simulink model "ZSPARK"  (R2026a)
settings: Solver=ode45  StopTime=0.010  FixedStep=1e-6
libraries: commrandsrc3 x5
settings Model: Creator=SANDESH  LastModifiedBy=SANDESH

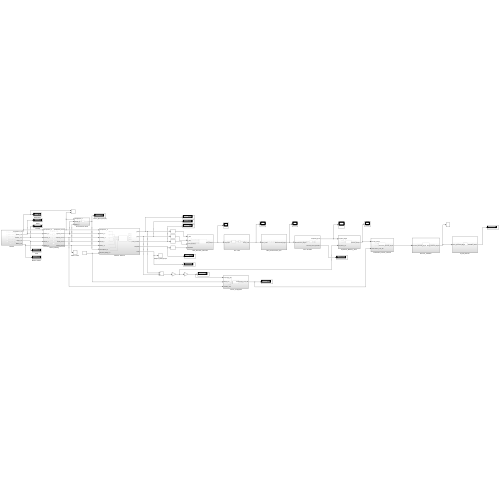
[thumbnail: Simulink's stored preview of the top-level diagram]
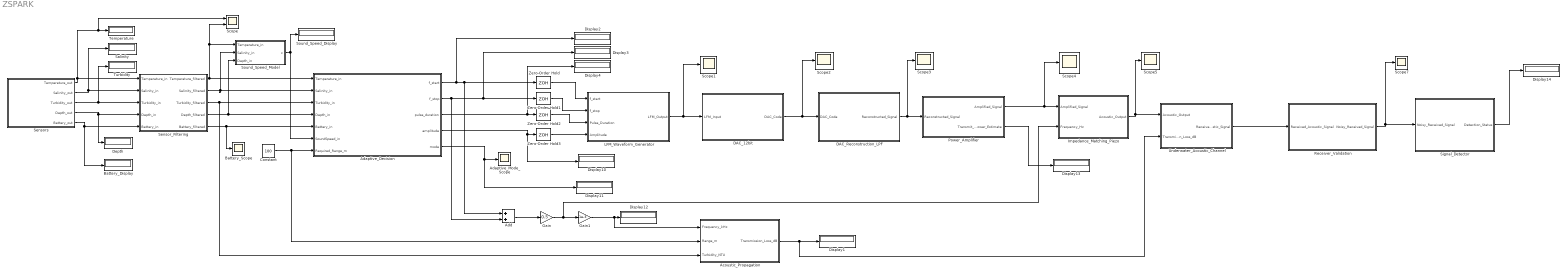
== system ZSPARK ==
  Acoustic_Propagation : Subsystem
  Adaptive_Decision : Subsystem
  Adaptive_Mode_Scope : Scope
      settings: TimeSpan=2  ActiveDisplayYMinimum=3  ActiveDisplayYMaximum=5  DataLoggingVariableName=ScopeData7
  Add : Sum
  Battery_Display : Display
  Battery_Scope : Scope
      settings: ActiveDisplayYMinimum=10.05  ActiveDisplayYMaximum=30.05  DataLoggingVariableName=ScopeData8
  Constant : Constant  Value=100
  DAC_12bit : Subsystem
  DAC_Reconstruction_LPF : Subsystem
  "Depth " : Display
  Display{1..4,10..14} (9 alike) : Display
  Gain : Gain  Gain=0.5
  Gain1 : Gain  Gain=1e-3
  Impedance_Matching_Piezo : Subsystem
  LFM_Waveform_Generator : Subsystem
  Power_Amplifier : Subsystem
  Receiver_Validation : Subsystem
  Salinity : Display
  Scope : Scope  NumInputPorts=2
      settings: TimeSpan=5  ActiveDisplayYMinimum=24.73062316838924  ActiveDisplayYMaximum=25.037041154016777
  Scope{1..5,7} (6 alike) : Scope
      Scope1 settings: TimeSpan=0.01  ActiveDisplayYMinimum=-1.0116208794215797  ActiveDisplayYMaximum=0.70243286352046441  DataLoggingDecimation=10
      Scope2 settings: TimeSpan=5e-3  ActiveDisplayYMinimum=1213.15  ActiveDisplayYMaximum=2904.4  DataLoggingVariableName=ScopeData2
      Scope3 settings: ActiveDisplayYMinimum=-0.37290125281823788  ActiveDisplayYMaximum=0.44819314690823536  DataLoggingVariableName=ScopeData3
      Scope4 settings: ActiveDisplayYMinimum=-0.82095317211603991  ActiveDisplayYMaximum=0.82123562733690658  DataLoggingVariableName=ScopeData4
      Scope5 settings: ActiveDisplayYMinimum=-0.38776131013108261  ActiveDisplayYMaximum=0.42690430214579189  DataLoggingVariableName=ScopeData5
      Scope7 settings: TimeSpan=0.01  ActiveDisplayYMinimum=-0.00440701448520266  ActiveDisplayYMaximum=0.0042196253860243855  DataLoggingVariableName=ScopeData9
  Sensor_Filtering : Subsystem
  Sensors : Subsystem
  Signal_Detector : Subsystem
  Sound_Speed_Display : Display
  Sound_Speed_Model : Subsystem
  "Temperature " : Display
  Turbidity : Display
  Underwater_Acoustic_Channel : Subsystem
  Zero-Order Hold{,1..3} (4 alike) : ZeroOrderHold  SampleTime=1e-6
  wires:
  Sensors/5(Battery_out) -> Sensor_Filtering/5(Battery_in), Battery_Display/1
  Sensors/4(Depth_out) -> Sensor_Filtering/4(Depth_in), "Depth "/1
  Sensors/2(Salinity_out) -> Sensor_Filtering/2(Salinity_in), Salinity/1
  Sensors/3("Turbidity_out ") -> Sensor_Filtering/3("Turbidity_in "), Turbidity/1
  Sensors/1(Temperature_out) -> Sensor_Filtering/1(Temperature_in), Scope/1, "Temperature "/1
  Sensor_Filtering/1(Temperature_filtered) -> Scope/2, Sound_Speed_Model/1(Temperature_in), Adaptive_Decision/1(Temperature_in)
  Sensor_Filtering/2(Salinity_filtered) -> Sound_Speed_Model/2(Salinity_in), Adaptive_Decision/2(Salinity_in)
  Sensor_Filtering/4(Depth_filtered) -> Sound_Speed_Model/3(Depth_in), Adaptive_Decision/4(Depth_in)
  Sound_Speed_Model/1(c) -> Adaptive_Decision/6(SoundSpeed_in), Sound_Speed_Display/1
  Gain1/1 -> Acoustic_Propagation/1(Frequency_kHz), Display12/1
  Constant/1 -> Acoustic_Propagation/2(Range_m), Adaptive_Decision/7(Required_Range_m)
  Sensor_Filtering/3(Turbidity_filtered) -> Acoustic_Propagation/3(Turbidity_NTU), Adaptive_Decision/3("Turbidity_in ")
  Sensor_Filtering/5(Battery_filtered) -> Battery_Scope/1, Adaptive_Decision/5(Battery_in)
  Adaptive_Decision/1(f_start) -> Display2/1, Add/1, Zero-Order Hold/1
  Adaptive_Decision/2(f_stop) -> Add/2, Zero-Order Hold1/1, Display3/1
  Adaptive_Decision/3(pulse_duration) -> Display4/1, Zero-Order Hold2/1
  Adaptive_Decision/5(mode) -> Display11/1, Adaptive_Mode_Scope/1
  Gain/1 -> Impedance_Matching_Piezo/2(Frequency_Hz), Gain1/1
  LFM_Waveform_Generator/1(LFM_Output) -> Scope1/1, DAC_12bit/1(LFM_Input)
  Zero-Order Hold/1 -> LFM_Waveform_Generator/1(f_start)
  Zero-Order Hold1/1 -> LFM_Waveform_Generator/2(f_stop)
  Zero-Order Hold3/1 -> LFM_Waveform_Generator/4(Amplitude)
  Zero-Order Hold2/1 -> LFM_Waveform_Generator/3(Pulse_Duration)
  DAC_12bit/1(DAC_Code) -> Scope2/1, DAC_Reconstruction_LPF/1(DAC_Code)
  DAC_Reconstruction_LPF/1(Reconstructed_Signal) -> Power_Amplifier/1(Reconstructed_Signal), Scope3/1
  Power_Amplifier/1(Amplified_Signal) -> Impedance_Matching_Piezo/1(Amplified_Signal), Scope4/1
  Power_Amplifier/2(Transmit_Power_Estimate) -> Display13/1
  Impedance_Matching_Piezo/1(Acoustic_Output) -> Scope5/1, Underwater_Acoustic_Channel/1(Acoustic_Output)
  Adaptive_Decision/4(amplitude) -> Display10/1, Zero-Order Hold3/1
  Add/1 -> Gain/1
  Underwater_Acoustic_Channel/1(Received_Acoustic_Signal) -> Receiver_Validation/1(Received_Acoustic_Signal)
  Acoustic_Propagation/1(Transmission_Loss_dB) -> Underwater_Acoustic_Channel/2(Transmission_Loss_dB), Display1/1
  Receiver_Validation/1(Noisy_Received_Signal) -> Signal_Detector/1(Noisy_Received_Signal), Scope7/1
  Signal_Detector/1(Detection_Status) -> Display14/1

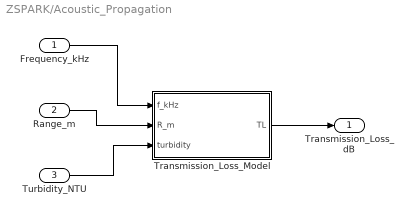
== system ZSPARK/Acoustic_Propagation ==
  Frequency_kHz : Inport
  Range_m : Inport  Port=2
  Turbidity_NTU : Inport  Port=3
  Transmission_Loss_Model : MATLAB Function  TreatAsAtomicUnit=on
  Transmission_Loss_dB : Outport
  wires:
  Frequency_kHz/1 -> Transmission_Loss_Model/1(f_kHz)
  Range_m/1 -> Transmission_Loss_Model/2(R_m)
  Turbidity_NTU/1 -> Transmission_Loss_Model/3(turbidity)
  Transmission_Loss_Model/1(TL) -> Transmission_Loss_dB/1

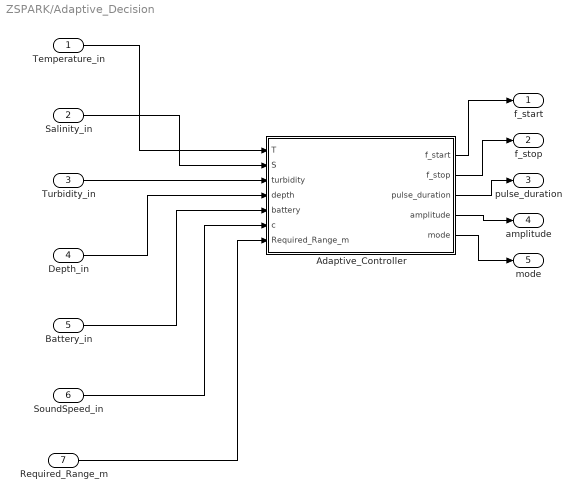
== system ZSPARK/Adaptive_Decision ==
  Temperature_in : Inport
  Salinity_in : Inport  Port=2
  "Turbidity_in " : Inport  Port=3
  Depth_in : Inport  Port=4
  Battery_in : Inport  Port=5
  SoundSpeed_in : Inport  Port=6
  Required_Range_m : Inport  Port=7
  Adaptive_Controller : MATLAB Function  TreatAsAtomicUnit=on
  f_start : Outport
  f_stop : Outport  Port=2
  pulse_duration : Outport  Port=3
  amplitude : Outport  Port=4
  mode : Outport  Port=5
  wires:
  Battery_in/1 -> Adaptive_Controller/5(battery)
  "Turbidity_in "/1 -> Adaptive_Controller/3(turbidity)
  Salinity_in/1 -> Adaptive_Controller/2(S)
  Temperature_in/1 -> Adaptive_Controller/1(T)
  Depth_in/1 -> Adaptive_Controller/4(depth)
  SoundSpeed_in/1 -> Adaptive_Controller/6(c)
  Adaptive_Controller/5(mode) -> mode/1
  Adaptive_Controller/4(amplitude) -> amplitude/1
  Adaptive_Controller/3(pulse_duration) -> pulse_duration/1
  Adaptive_Controller/2(f_stop) -> f_stop/1
  Adaptive_Controller/1(f_start) -> f_start/1
  Required_Range_m/1 -> Adaptive_Controller/7(Required_Range_m)

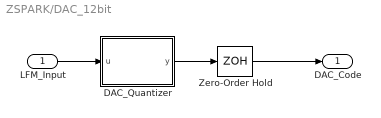
== system ZSPARK/DAC_12bit ==
  LFM_Input : Inport
  DAC_Quantizer : MATLAB Function  TreatAsAtomicUnit=on
  Zero-Order Hold : ZeroOrderHold  SampleTime=-1
  DAC_Code : Outport
  wires:
  LFM_Input/1 -> DAC_Quantizer/1(u)
  DAC_Quantizer/1(y) -> Zero-Order Hold/1
  Zero-Order Hold/1 -> DAC_Code/1

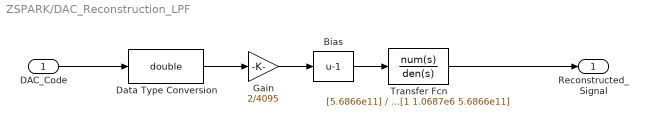
== system ZSPARK/DAC_Reconstruction_LPF ==
  DAC_Code : Inport
  Bias : Bias  Bias=-1  SaturateOnIntegerOverflow=off
  Data Type Conversion : DataTypeConversion  OutDataTypeStr=double  SaturateOnIntegerOverflow=off  RndMeth=Floor
  Gain : Gain  Gain=2/4095
  Transfer Fcn : TransferFcn  Numerator=[5.6866e11]  Denominator=[1 1.0687e6 5.6866e11]
  Reconstructed_Signal : Outport
  wires:
  DAC_Code/1 -> Data Type Conversion/1
  Data Type Conversion/1 -> Gain/1
  Gain/1 -> Bias/1
  Bias/1 -> Transfer Fcn/1
  Transfer Fcn/1 -> Reconstructed_Signal/1

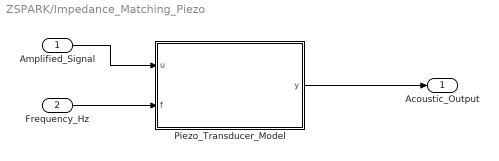
== system ZSPARK/Impedance_Matching_Piezo ==
  Amplified_Signal : Inport
  Frequency_Hz : Inport  Port=2
  Piezo_Transducer_Model : MATLAB Function  TreatAsAtomicUnit=on
  Acoustic_Output : Outport
  wires:
  Frequency_Hz/1 -> Piezo_Transducer_Model/2(f)
  Amplified_Signal/1 -> Piezo_Transducer_Model/1(u)
  Piezo_Transducer_Model/1(y) -> Acoustic_Output/1

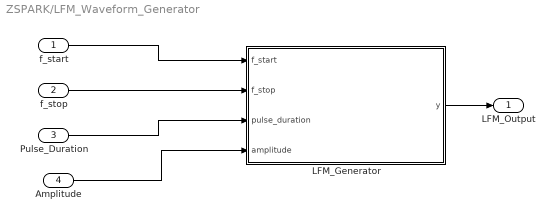
== system ZSPARK/LFM_Waveform_Generator ==
  f_start : Inport
  f_stop : Inport  Port=2
  Pulse_Duration : Inport  Port=3
  Amplitude : Inport  Port=4
  LFM_Generator : MATLAB Function  TreatAsAtomicUnit=on
  LFM_Output : Outport
  wires:
  f_start/1 -> LFM_Generator/1(f_start)
  f_stop/1 -> LFM_Generator/2(f_stop)
  Pulse_Duration/1 -> LFM_Generator/3(pulse_duration)
  Amplitude/1 -> LFM_Generator/4(amplitude)
  LFM_Generator/1(y) -> LFM_Output/1

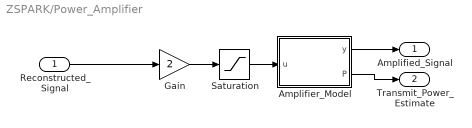
== system ZSPARK/Power_Amplifier ==
  Reconstructed_Signal : Inport
  Amplifier_Model : MATLAB Function  TreatAsAtomicUnit=on
  Gain : Gain  Gain=2
  Saturation : Saturate  UpperLimit=1  LowerLimit=-1
  Amplified_Signal : Outport
  Transmit_Power_Estimate : Outport  Port=2
  wires:
  Reconstructed_Signal/1 -> Gain/1
  Gain/1 -> Saturation/1
  Saturation/1 -> Amplifier_Model/1(u)
  Amplifier_Model/1(y) -> Amplified_Signal/1
  Amplifier_Model/2(P) -> Transmit_Power_Estimate/1

== system ZSPARK/Receiver_Validation ==
  Received_Acoustic_Signal : Inport
  Underwater_Noise_Model : MATLAB Function  TreatAsAtomicUnit=on
  Noisy_Received_Signal : Outport
  wires:
  Received_Acoustic_Signal/1 -> Underwater_Noise_Model/1(u)
  Underwater_Noise_Model/1(y) -> Noisy_Received_Signal/1

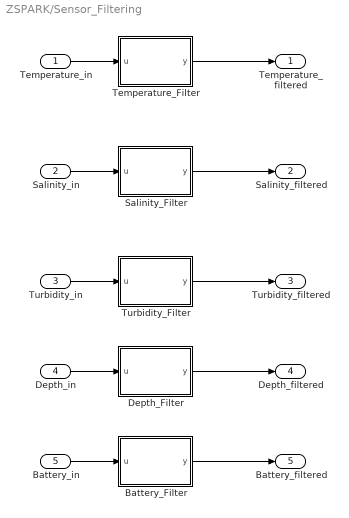
== system ZSPARK/Sensor_Filtering ==
  Temperature_in : Inport
  Salinity_in : Inport  Port=2
  "Turbidity_in " : Inport  Port=3
  Depth_in : Inport  Port=4
  Battery_in : Inport  Port=5
  Battery_Filter : MATLAB Function  TreatAsAtomicUnit=on
  Depth_Filter : MATLAB Function  TreatAsAtomicUnit=on
  Salinity_Filter : MATLAB Function  TreatAsAtomicUnit=on
  "Temperature_Filter " : MATLAB Function  TreatAsAtomicUnit=on
  Turbidity_Filter : MATLAB Function  TreatAsAtomicUnit=on
  Temperature_filtered : Outport
  Salinity_filtered : Outport  Port=2
  Turbidity_filtered : Outport  Port=3
  Depth_filtered : Outport  Port=4
  Battery_filtered : Outport  Port=5
  wires:
  Temperature_in/1 -> "Temperature_Filter "/1(u)
  Salinity_in/1 -> Salinity_Filter/1(u)
  "Turbidity_in "/1 -> Turbidity_Filter/1(u)
  Depth_in/1 -> Depth_Filter/1(u)
  Battery_in/1 -> Battery_Filter/1(u)
  "Temperature_Filter "/1(y) -> Temperature_filtered/1
  Salinity_Filter/1(y) -> Salinity_filtered/1
  Turbidity_Filter/1(y) -> Turbidity_filtered/1
  Depth_Filter/1(y) -> Depth_filtered/1
  Battery_Filter/1(y) -> Battery_filtered/1

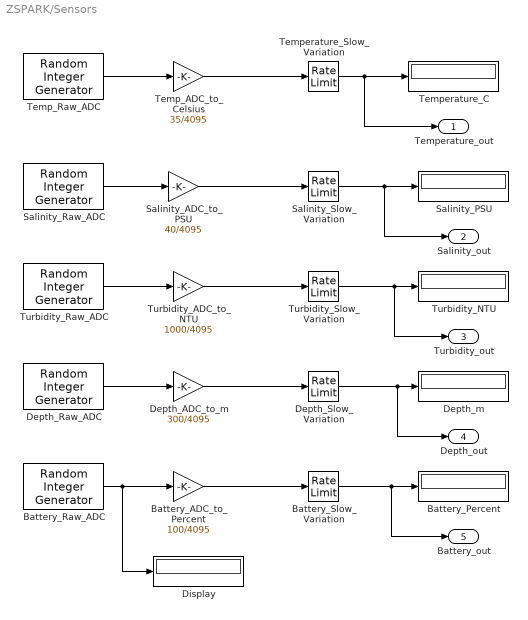
== system ZSPARK/Sensors ==
  Battery_ADC_to_Percent : Gain  Gain=100/4095
  Battery_Percent : Display
  Battery_Raw_ADC : commrandsrc3/Random Integer Generator  SetSize=4096  SeedSource=Parameter  Seed=56789  SampleTime=0.1  SamplesPerFrame=1  OutputDataType=double  SimulateUsing=Interpreted execution
  Battery_Slow_Variation : RateLimiter  RisingSlewLimit=0.5  FallingSlewLimit=-0.5  SampleTimeMode=inherited  InitialCondition=20
  Depth_ADC_to_m : Gain  Gain=300/4095
  Depth_Raw_ADC : commrandsrc3/Random Integer Generator  SetSize=2730  SeedSource=Parameter  Seed=45678  SampleTime=0.1  SamplesPerFrame=1  OutputDataType=double  SimulateUsing=Interpreted execution
  Depth_Slow_Variation : RateLimiter  RisingSlewLimit=2  FallingSlewLimit=-2  SampleTimeMode=inherited  InitialCondition=100
  Depth_m : Display
  Display : Display
  Salinity_ADC_to_PSU : Gain  Gain=40/4095
  Salinity_PSU : Display
  Salinity_Raw_ADC : commrandsrc3/Random Integer Generator  SetSize=4096  SeedSource=Parameter  Seed=23456  SampleTime=0.1  SamplesPerFrame=1  OutputDataType=double  SimulateUsing=Interpreted execution
  Salinity_Slow_Variation : RateLimiter  RisingSlewLimit=0.2  FallingSlewLimit=-0.2  SampleTimeMode=inherited  InitialCondition=35
  Temp_ADC_to_Celsius : Gain  Gain=35/4095
  Temp_Raw_ADC : commrandsrc3/Random Integer Generator  SetSize=4096  SeedSource=Parameter  Seed=12345  SampleTime=0.1  SamplesPerFrame=1  OutputDataType=double  SimulateUsing=Interpreted execution
  Temperature_C : Display
  Temperature_Slow_Variation : RateLimiter  RisingSlewLimit=0.2  FallingSlewLimit=-0.2  SampleTimeMode=inherited  InitialCondition=25
  Turbidity_ADC_to_NTU : Gain  Gain=1000/4095
  Turbidity_NTU : Display
  Turbidity_Raw_ADC : commrandsrc3/Random Integer Generator  SetSize=4096  SeedSource=Parameter  Seed=34567  SampleTime=0.1  SamplesPerFrame=1  OutputDataType=double  SimulateUsing=Interpreted execution
  Turbidity_Slow_Variation : RateLimiter  RisingSlewLimit=20  FallingSlewLimit=-20  SampleTimeMode=inherited  InitialCondition=500
  Temperature_out : Outport
  Salinity_out : Outport  Port=2
  "Turbidity_out " : Outport  Port=3
  Depth_out : Outport  Port=4
  Battery_out : Outport  Port=5
  wires:
  Temp_Raw_ADC/1 -> Temp_ADC_to_Celsius/1
  Salinity_Raw_ADC/1 -> Salinity_ADC_to_PSU/1
  Turbidity_Raw_ADC/1 -> Turbidity_ADC_to_NTU/1
  Depth_Raw_ADC/1 -> Depth_ADC_to_m/1
  Battery_Raw_ADC/1 -> Display/1, Battery_ADC_to_Percent/1
  Temp_ADC_to_Celsius/1 -> Temperature_Slow_Variation/1
  Temperature_Slow_Variation/1 -> Temperature_out/1, Temperature_C/1
  Salinity_ADC_to_PSU/1 -> Salinity_Slow_Variation/1
  Salinity_Slow_Variation/1 -> Salinity_out/1, Salinity_PSU/1
  Turbidity_ADC_to_NTU/1 -> Turbidity_Slow_Variation/1
  Turbidity_Slow_Variation/1 -> "Turbidity_out "/1, Turbidity_NTU/1
  Depth_ADC_to_m/1 -> Depth_Slow_Variation/1
  Depth_Slow_Variation/1 -> Depth_out/1, Depth_m/1
  Battery_Slow_Variation/1 -> Battery_out/1, Battery_Percent/1
  Battery_ADC_to_Percent/1 -> Battery_Slow_Variation/1

== system ZSPARK/Signal_Detector ==
  Noisy_Received_Signal : Inport
  Echo_Detector : MATLAB Function  TreatAsAtomicUnit=on
  Detection_Status : Outport
  wires:
  Noisy_Received_Signal/1 -> Echo_Detector/1(u)
  Echo_Detector/1(detected) -> Detection_Status/1

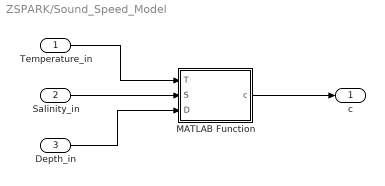
== system ZSPARK/Sound_Speed_Model ==
  Temperature_in : Inport
  Salinity_in : Inport  Port=2
  Depth_in : Inport  Port=3
  MATLAB Function : MATLAB Function  TreatAsAtomicUnit=on
  c : Outport
  wires:
  Salinity_in/1 -> MATLAB Function/2(S)
  Depth_in/1 -> MATLAB Function/3(D)
  Temperature_in/1 -> MATLAB Function/1(T)
  MATLAB Function/1(c) -> c/1

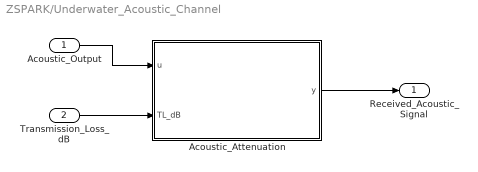
== system ZSPARK/Underwater_Acoustic_Channel ==
  Acoustic_Output : Inport
  Transmission_Loss_dB : Inport  Port=2
  Acoustic_Attenuation : MATLAB Function  TreatAsAtomicUnit=on
  Received_Acoustic_Signal : Outport
  wires:
  Acoustic_Output/1 -> Acoustic_Attenuation/1(u)
  Transmission_Loss_dB/1 -> Acoustic_Attenuation/2(TL_dB)
  Acoustic_Attenuation/1(y) -> Received_Acoustic_Signal/1

== matlab function ZSPARK/Power_Amplifier/Amplifier_Model ==
  data: u input; y output; P output
function [y,P] = fcn(u)

% Simple transmitter amplifier model
% u = amplifier input signal

% Amplifier enable
enable = 1;

% Approximate output signal
if enable == 1
    y = u;
else
    y = 0;
end

% Relative transmit power estimate
P = y*y;

end

== matlab function ZSPARK/Impedance_Matching_Piezo/Piezo_Transducer_Model ==
  data: u input; y output; f input
function y = fcn(u,f)

% =========================================================
% IMPEDANCE MATCHING + PIEZOELECTRIC TRANSDUCER MODEL
% =========================================================

% Nominal transducer frequency
f0 = 60e3;

% Approximate transducer bandwidth
BW = 35e3;

% Frequency offset from resonance
df = f - f0;

% Normalized frequency response
H = 1 / sqrt(1 + (2*df/BW)^2);

% Approximate impedance-matching efficiency
eta_match = 0.85;

% Overall acoustic conversion factor
conversion = 0.75;

% Final acoustic output
y = u * H * eta_match * conversion;

end

== matlab function ZSPARK/Underwater_Acoustic_Channel/Acoustic_Attenuation ==
  data: u input; y output; TL_dB input
function y = fcn(u,TL_dB)

% =========================================================
% UNDERWATER ACOUSTIC PROPAGATION
% =========================================================
% u     = acoustic transmit signal
% TL_dB = transmission loss in dB
%
% Amplitude attenuation:
%
%       A = 10^(-TL/20)
%
% =========================================================

TL_dB = max(TL_dB,0);

attenuation = 10^(-TL_dB/20);

y = u * attenuation;

end

== matlab function ZSPARK/Receiver_Validation/Underwater_Noise_Model ==
  settings: updateMethod=DISCRETE
  data: u input; y output
function y = fcn(u)

% ==========================================
% UNDERWATER RECEIVER NOISE MODEL
% ==========================================

% Noise level for simulation
noise_std = 0.0005;

% Generate underwater/background noise
noise = noise_std * randn;

% Received signal + noise
y = u + noise;

end

== matlab function ZSPARK/Signal_Detector/Echo_Detector ==
  data: u input; detected output
function detected = fcn(u)

% Simple energy-based sonar detector

persistent energy

if isempty(energy)
    energy = 0;
end

% Smooth signal energy
alpha = 0.01;
energy = (1-alpha)*energy + alpha*(u*u);

% Detection threshold
threshold = 1e-7;

if energy > threshold
    detected = 1;
else
    detected = 0;
end

end

== matlab function ZSPARK/Sensor_Filtering/Salinity_Filter ==
  data: u input; y output
function y = fcn(u)

persistent buffer count

if isempty(buffer)
    buffer = zeros(1,10);
    count = 0;
end

if count < 10
    count = count + 1;
    buffer(count) = u;
    y = mean(buffer(1:count));
else
    y = mean(buffer);
    buffer = [buffer(2:end) u];
end

end

== matlab function ZSPARK/Sensor_Filtering/Temperature_Filter  ==
  data: u input; y output
function y = fcn(u)

persistent buffer count

if isempty(buffer)
    buffer = zeros(1,10);
    count = 0;
end

if count < 10
    count = count + 1;
    buffer(count) = u;
    y = mean(buffer(1:count));
else
    y = mean(buffer);
    buffer = [buffer(2:end) u];
end

end

== matlab function ZSPARK/Sensor_Filtering/Turbidity_Filter ==
  data: u input; y output
function y = fcn(u)

persistent buffer count

if isempty(buffer)
    buffer = zeros(1,10);
    count = 0;
end

if count < 10
    count = count + 1;
    buffer(count) = u;
    y = mean(buffer(1:count));
else
    y = mean(buffer);
    buffer = [buffer(2:end) u];
end

end

== matlab function ZSPARK/Sensor_Filtering/Depth_Filter ==
  data: u input; y output
function y = fcn(u)

persistent buffer count

if isempty(buffer)
    buffer = zeros(1,10);
    count = 0;
end

if count < 10
    count = count + 1;
    buffer(count) = u;
    y = mean(buffer(1:count));
else
    y = mean(buffer);
    buffer = [buffer(2:end) u];
end

end

== matlab function ZSPARK/Sensor_Filtering/Battery_Filter ==
  data: u input; y output
function y = fcn(u)

persistent buffer count

if isempty(buffer)
    buffer = zeros(1,10);
    count = 0;
end

if count < 10
    count = count + 1;
    buffer(count) = u;
    y = mean(buffer(1:count));
else
    y = mean(buffer);
    buffer = [buffer(2:end) u];
end

end

== matlab function ZSPARK/Sound_Speed_Model/MATLAB Function ==
  data: T input; c output; S input; D input
function c = fcn(T,S,D)

% Keep inputs within Mackenzie equation validity range
T = min(max(T,2),30);
S = min(max(S,25),40);
D = min(max(D,0),8000);

% Mackenzie sound-speed equation
c = 1448.96 ...
    + 4.591*T ...
    - 5.304e-2*T^2 ...
    + 2.374e-4*T^3 ...
    + 1.340*(S-35) ...
    + 1.630e-2*D ...
    + 1.675e-7*D^2 ...
    - 1.025e-2*T*(S-35) ...
    - 7.139e-13*T*D^3;

end

== matlab function ZSPARK/Acoustic_Propagation/Transmission_Loss_Model ==
  data: f_kHz input; TL output; R_m input; turbidity input
function TL = fcn(f_kHz, R_m, turbidity)

% Prevent invalid values
f_kHz = max(f_kHz,0.1);
R_m   = max(R_m,1);
turbidity = max(turbidity,0);

% ------------------------------------------------
% 1. Spherical spreading loss
% ------------------------------------------------
SpreadingLoss = 20*log10(R_m);

% ------------------------------------------------
% 2. Thorp absorption coefficient
%    f is in kHz
%    alpha is approximately dB/km
% ------------------------------------------------
alpha = 0.11*(f_kHz^2)/(1 + f_kHz^2) ...
      + 44*(f_kHz^2)/(4100 + f_kHz^2) ...
      + 2.75e-4*(f_kHz^2) ...
      + 0.003;

% Convert range from m to km
R_km = R_m/1000;

% Absorption loss
AbsorptionLoss = alpha*R_km;

% ------------------------------------------------
% 3. Simple empirical turbidity/scattering term
% ------------------------------------------------
% This is a simulation tuning term, NOT a universal
% physical turbidity law.
TurbidityLoss = 0.005*turbidity*R_km;

% ------------------------------------------------
% Total transmission loss
% ------------------------------------------------
TL = SpreadingLoss + AbsorptionLoss + TurbidityLoss;

end

== matlab function ZSPARK/Adaptive_Decision/Adaptive_Controller ==
  data: T input; f_start output; S input; turbidity input; depth input; battery input; c input; f_stop output; pulse_duration output; amplitude output; mode output; Required_Range_m input
function [f_start,f_stop,pulse_duration,amplitude,mode] = ...
    fcn(T,S,turbidity,depth,battery,c,Required_Range_m)

% =========================================================
% SPARKX ADAPTIVE SONAR DECISION ENGINE
% =========================================================
%
% Inputs:
% T                 Temperature (deg C)
% S                 Salinity (PSU)
% turbidity         Turbidity (NTU)
% depth             AUV depth (m)
% battery           Battery level (%)
% c                 Sound speed (m/s)
% Required_Range_m  Required sonar target range (m)
%
% Outputs:
% f_start           LFM starting frequency (Hz)
% f_stop            LFM stopping frequency (Hz)
% pulse_duration    Pulse duration (s)
% amplitude         Normalized transmit amplitude
% mode              Selected operating mode
%
% Three candidate operating bands:
%
% Mode 1 = High-resolution
% Mode 2 = Balanced
% Mode 3 = Long-range / difficult environment
%
% Mode 4 = Low-battery protection
%
% =========================================================

% ---------------------------------------------------------
% Safety limits
% ---------------------------------------------------------

T = min(max(T,2),30);
S = min(max(S,25),40);
turbidity = max(turbidity,0);
depth = max(depth,0);
battery = min(max(battery,0),100);
c = max(c,1400);
Required_Range_m = max(Required_Range_m,10);

% ---------------------------------------------------------
% Persistent mode provides hysteresis
% ---------------------------------------------------------

persistent previous_mode

if isempty(previous_mode)
    previous_mode = 2;
end

% ---------------------------------------------------------
% Candidate frequency bands
% ---------------------------------------------------------

start_kHz = [40 30 20];
stop_kHz  = [100 70 50];

% Pulse durations for the three candidates
pulse_candidates = [6e-3 10e-3 15e-3];

% Base amplitudes
amp_candidates = [0.55 0.60 0.65];

% ---------------------------------------------------------
% Environment severity
% ---------------------------------------------------------

turbidity_index = min(turbidity/1000,1);

depth_index = min(depth/300,1);

range_index = min(Required_Range_m/300,1);

battery_stress = 1 - battery/100;

% ---------------------------------------------------------
% Calculate score for each candidate
% Lower score = better choice
% ---------------------------------------------------------

score = zeros(1,3);

for i = 1:3

    % Center frequency
    center_kHz = (start_kHz(i)+stop_kHz(i))/2;

    % Bandwidth
    bandwidth_Hz = (stop_kHz(i)-start_kHz(i))*1000;

    % LFM range resolution
    resolution_m = c/(2*bandwidth_Hz);

    % -----------------------------------------------------
    % Estimated propagation loss
    % -----------------------------------------------------

    f = center_kHz;
    R = Required_Range_m;

    spreading_loss = 20*log10(R);

    alpha = 0.11*(f^2)/(1+f^2) ...
          + 44*(f^2)/(4100+f^2) ...
          + 2.75e-4*(f^2) ...
          + 0.003;

    absorption_loss = alpha*(R/1000);

    turbidity_loss = 0.005*turbidity*(R/1000);

    total_loss = spreading_loss ...
               + absorption_loss ...
               + turbidity_loss;

    % -----------------------------------------------------
    % Normalize propagation loss
    % -----------------------------------------------------

    loss_index = min(total_loss/70,1);

    % -----------------------------------------------------
    % Resolution cost
    % Smaller resolution is better
    % -----------------------------------------------------

    resolution_index = min(resolution_m/Required_Range_m,1);

    % -----------------------------------------------------
    % Energy cost
    % Approximate relative transmit energy
    % -----------------------------------------------------

    energy_index = amp_candidates(i)^2 ...
                 * pulse_candidates(i)/15e-3;

    % -----------------------------------------------------
    % Environment penalty
    %
    % Higher frequency is penalized in difficult water
    % -----------------------------------------------------

    if i == 1
        high_frequency_penalty = ...
            0.50*turbidity_index + ...
            0.20*range_index;
    elseif i == 2
        high_frequency_penalty = ...
            0.20*turbidity_index + ...
            0.10*range_index;
    else
        high_frequency_penalty = 0;
    end

    % -----------------------------------------------------
    % Battery penalty
    % -----------------------------------------------------

    battery_penalty = battery_stress*energy_index;

    % -----------------------------------------------------
    % Final candidate score
    % -----------------------------------------------------

    score(i) = ...
        0.40*loss_index + ...
        0.25*resolution_index + ...
        0.15*energy_index + ...
        0.20*high_frequency_penalty + ...
        0.20*battery_penalty;

end

% ---------------------------------------------------------
% Find best candidate
% ---------------------------------------------------------

[~,best_mode] = min(score);

% ---------------------------------------------------------
% Hysteresis
% Do not change mode for tiny score differences
% ---------------------------------------------------------

hysteresis = 0.05;

if best_mode ~= previous_mode

    if score(best_mode) + hysteresis < score(previous_mode)
        previous_mode = best_mode;
    end

end

mode = previous_mode;

% ---------------------------------------------------------
% Low-battery protection
% ---------------------------------------------------------

if battery < 25

    mode = 4;

end

% ---------------------------------------------------------
% Select frequency and basic pulse parameters
% ---------------------------------------------------------

if mode == 1

    % High resolution
    f_start = 40e3;
    f_stop = 100e3;

    pulse_duration = 6e-3;
    amplitude = 0.55;

elseif mode == 2

    % Balanced operation
    f_start = 30e3;
    f_stop = 70e3;

    pulse_duration = 10e-3;
    amplitude = 0.60;

elseif mode == 3

    % Long-range / difficult environment
    f_start = 20e3;
    f_stop = 50e3;

    pulse_duration = 15e-3;
    amplitude = 0.65;

else

    % Low-battery protection
    f_start = 20e3;
    f_stop = 50e3;

    pulse_duration = 5e-3;
    amplitude = 0.40;

end

% ---------------------------------------------------------
% Adaptive amplitude based on propagation difficulty
% ---------------------------------------------------------

center_kHz = (f_start + f_stop)/2000;

spreading_loss = 20*log10(Required_Range_m);

alpha = 0.11*(center_kHz^2)/(1+center_kHz^2) ...
      + 44*(center_kHz^2)/(4100+center_kHz^2) ...
      + 2.75e-4*(center_kHz^2) ...
      + 0.003;

absorption_loss = alpha*(Required_Range_m/1000);

turbidity_loss = ...
    0.005*turbidity*(Required_Range_m/1000);

total_loss = spreading_loss ...
           + absorption_loss ...
           + turbidity_loss;

loss_index = min(total_loss/70,1);

% Increase amplitude only when propagation is difficult
amplitude = amplitude + 0.10*loss_index;

% ---------------------------------------------------------
% Battery protection
% ---------------------------------------------------------

if battery < 50
    amplitude = amplitude*0.90;
end

if battery < 35
    amplitude = amplitude*0.80;
end

% ---------------------------------------------------------
% Final amplitude limit
% ---------------------------------------------------------

amplitude = min(max(amplitude,0.30),0.85);

end

== matlab function ZSPARK/LFM_Waveform_Generator/LFM_Generator ==
  data: f_start input; y output; f_stop input; pulse_duration input; amplitude input
function y = fcn(f_start,f_stop,pulse_duration,amplitude)

% =========================================================
% SAMPLE-BY-SAMPLE LFM SONAR GENERATOR
% =========================================================

Fs = 1e6;

persistent n

if isempty(n)
    n = 0;
end

% ---------------------------------------------------------
% Safety limits
% ---------------------------------------------------------

f_start = max(f_start,1e3);
f_stop = max(f_stop,f_start);

pulse_duration = min(max(pulse_duration,1e-3),20e-3);

amplitude = min(max(amplitude,0),1);

% Number of samples in pulse
N = round(Fs*pulse_duration);

% ---------------------------------------------------------
% Generate one sample
% ---------------------------------------------------------

if n < N

    t = n/Fs;

    k = (f_stop-f_start)/pulse_duration;

    phase = 2*pi*(f_start*t + 0.5*k*t*t);

    % Hann window
    if N > 1
        window = 0.5*(1-cos(2*pi*n/(N-1)));
    else
        window = 1;
    end

    y = amplitude*cos(phase)*window;

    n = n + 1;

else

    y = 0;

    n = 0;

end

end

== matlab function ZSPARK/DAC_12bit/DAC_Quantizer ==
  data: u input; y output
function y = fcn(u)

% =========================================================
% 12-BIT DAC QUANTIZER
% =========================================================
% Input:
%   u = normalized signal from -1 to +1
%
% Output:
%   y = 12-bit unsigned DAC code
%
% DAC range:
%   0 to 4095
% =========================================================

% Limit input to DAC range
u = min(max(u,-1),1);

% Convert -1...+1 to 0...4095
code = ((u + 1)/2)*4095;

% Quantize
code = round(code);

% Output as unsigned 12-bit-compatible value
y = uint16(code);

end
